simulink model "velocity"  (R2019a)
settings: Solver=ode45  StartTime=0.0  StopTime=3  MaxStep=0.0001  RelTol=1e-3
settings Model: Creator=ChairmanYang1966  LastModifiedBy=ChairmanYang1966

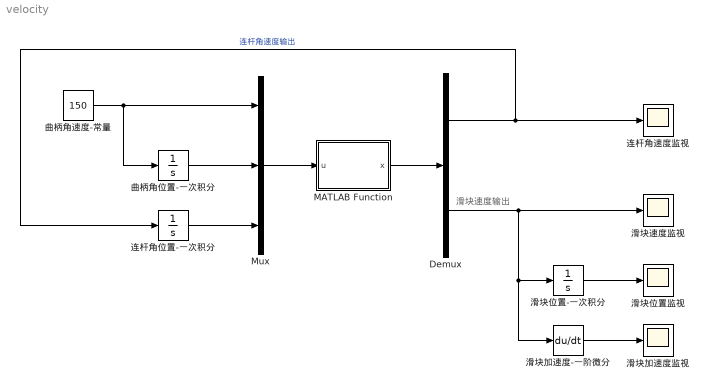
== system velocity ==
  note: 滑块速度输出
  Demux : Demux  Outputs=2
  MATLAB Function : MATLAB Function  TreatAsAtomicUnit=on
  Mux : Mux  Inputs=3
  曲柄角位置-一次积分 : Integrator
  曲柄角速度-常量 : Constant  Value=150
  滑块位置-一次积分 : Integrator  InitialCondition=70
  滑块位置监视 : Scope
  滑块加速度-一阶微分 : Derivative
  滑块加速度监视 : Scope
  滑块速度监视 : Scope
  连杆角位置-一次积分 : Integrator
  连杆角速度监视 : Scope
  wires:
  Mux/1 -> MATLAB Function/1(u)
  MATLAB Function/1(x) -> Demux/1
  曲柄角速度-常量/1 -> 曲柄角位置-一次积分/1, Mux/1
  曲柄角位置-一次积分/1 -> Mux/2
  Demux/2 -> 滑块加速度-一阶微分/1, 滑块位置-一次积分/1, 滑块速度监视/1
  滑块位置-一次积分/1 -> 滑块位置监视/1
  滑块加速度-一阶微分/1 -> 滑块加速度监视/1
  Demux/1 -> 连杆角位置-一次积分/1, 连杆角速度监视/1  "连杆角速度输出"
  连杆角位置-一次积分/1 -> Mux/3

== matlab function velocity/MATLAB Function ==
  data: u input; x output
function x = compv(u)
r1=15;r2=55;
x=[0;0];
a=[r2*sin(u(3)) 1;r2*cos(u(3)) 0];
b=-u(1)*r1*[sin(u(2));cos(u(2))];
x = inv(a)*b;
%曲柄长15mm，连杆长55mm
%u(1)指征曲柄角速度，u(2)指征曲柄角位置，u(3)指示连杆角位置
%x(1)指征连杆角速度，x(2)指征滑块加速度
